simulink model "ADC_SPWM_Openloop_2_Version_2"  (R2024b)
settings: Solver=FixedStepDiscrete  StartTime=0.0  StopTime=inf  FixedStep=50e-6  RelTol=1e-3
model workspace (MAT data in the model file):
  f = 25
undefined symbols (not defined in the file): alpha, alpha_Lpf, C28x, CPU1, CPU2, DiscIntNeverNeededParam, Down, dspblkCoreblockFVToolHelper, Gain, gcbh, GPTRIP1SEL, T_period, Ts, TZ1, Up
libraries: c2802xlib x26, dspstat3 x8, c2837xDlib x2, c280xlib x2, simulink x1, mcbpositiondecoderlib x1, mcbcontrolslib x1
(part 2 of 2)

== system ADC_SPWM_Openloop_2_Version_2/If Action Subsystem ==
  In1 : Inport
  Action Port : ActionPort  ActionPortLabel=if(u1 > 0.005)
  Out1 : Outport
  wires:
  In1/1 -> Out1/1

== system ADC_SPWM_Openloop_2_Version_2/If Action Subsystem1 ==
  In1 : Inport
  Action Port : ActionPort  ActionPortLabel=else
  Gain : Gain  Gain=0
  Out1 : Outport
  wires:
  In1/1 -> Gain/1
  Gain/1 -> Out1/1

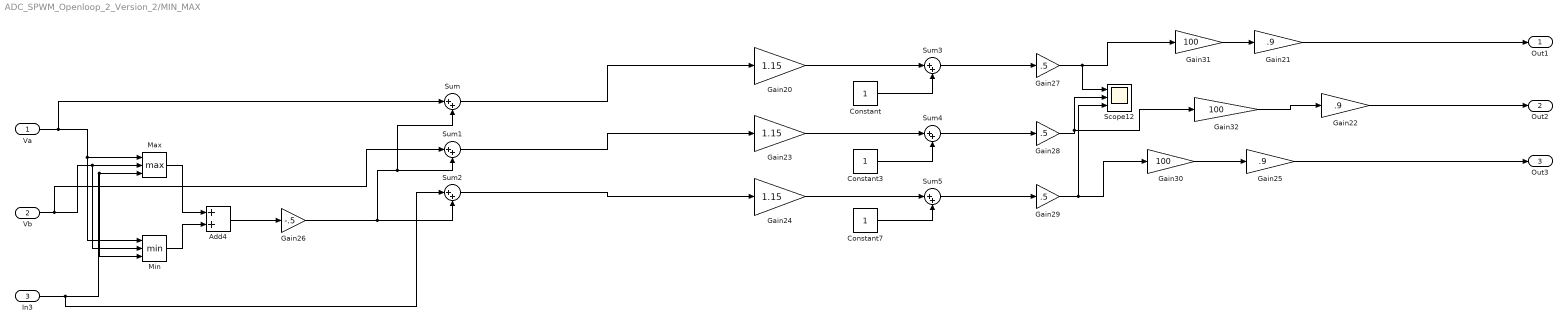
== system ADC_SPWM_Openloop_2_Version_2/MIN_MAX ==
  Va : Inport
  Vb : Inport  Port=2
  In3 : Inport  Port=3
  Add4 : Sum
  Constant : Constant
  Constant3 : Constant
  Constant7 : Constant
  Gain20 : Gain  Gain=1.15
  Gain21 : Gain  Gain=.9
  Gain22 : Gain  Gain=.9
  Gain23 : Gain  Gain=1.15
  Gain24 : Gain  Gain=1.15
  Gain25 : Gain  Gain=.9
  Gain26 : Gain  Gain=-.5
  Gain27 : Gain  Gain=.5
  Gain28 : Gain  Gain=.5
  Gain29 : Gain  Gain=.5
  Gain30 : Gain  Gain=100
  Gain31 : Gain  Gain=100
  Gain32 : Gain  Gain=100
  Max : MinMax  Function=max  Inputs=3
  Min : MinMax  Inputs=3
  Scope12 : Scope  NumInputPorts=3
  Sum{,1..5} (6 alike) : Sum  Inputs=|++
  Out1 : Outport
  Out2 : Outport  Port=2
  Out3 : Outport  Port=3
  wires:
  Gain28/1 -> Scope12/2, Gain32/1
  Sum3/1 -> Gain27/1
  Va/1 -> Sum/1, Min/1, Max/1
  Gain32/1 -> Gain22/1
  In3/1 -> Sum2/1, Min/3, Max/3
  Gain29/1 -> Scope12/3, Gain30/1
  Vb/1 -> Sum1/1, Min/2, Max/2
  Constant7/1 -> Sum5/2
  Sum/1 -> Gain20/1
  Gain26/1 -> Sum/2, Sum1/2, Sum2/2
  Add4/1 -> Gain26/1
  Gain30/1 -> Gain25/1
  Min/1 -> Add4/2
  Gain20/1 -> Sum3/1
  Gain27/1 -> Scope12/1, Gain31/1
  Constant3/1 -> Sum4/2
  Gain24/1 -> Sum5/1
  Constant/1 -> Sum3/2
  Sum4/1 -> Gain28/1
  Gain21/1 -> Out1/1
  Sum1/1 -> Gain23/1
  Max/1 -> Add4/1
  Gain25/1 -> Out3/1
  Gain31/1 -> Gain21/1
  Sum2/1 -> Gain24/1
  Gain23/1 -> Sum4/1
  Sum5/1 -> Gain29/1
  Gain22/1 -> Out2/1

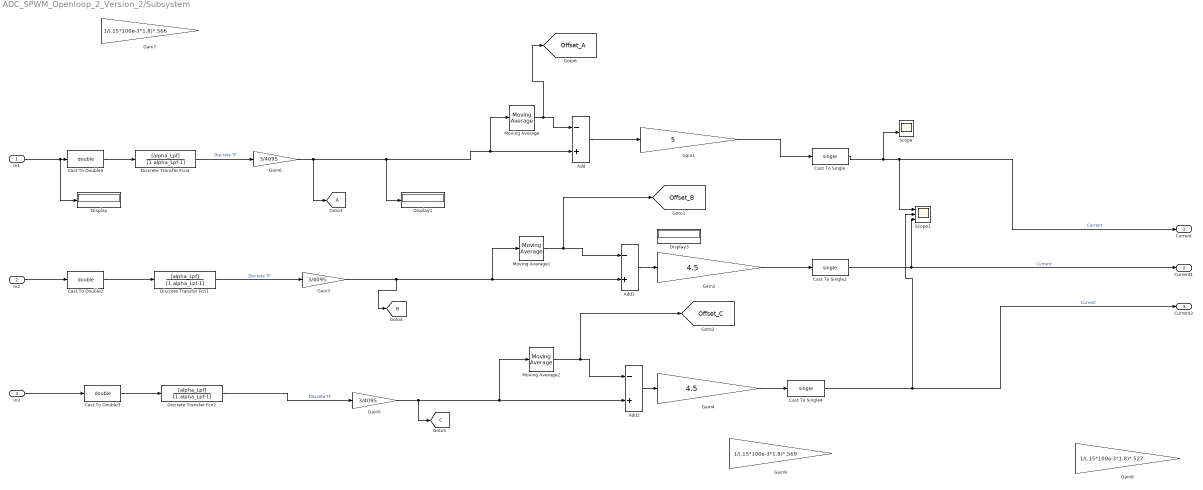
== system ADC_SPWM_Openloop_2_Version_2/Subsystem ==
  In1 : Inport
  In2 : Inport  Port=2
  In3 : Inport  Port=3
  Add : Sum  Inputs=-+
  Add1 : Sum  Inputs=-+
  Add2 : Sum  Inputs=-+
  Cast To Double2 : DataTypeConversion  OutDataTypeStr=double  SaturateOnIntegerOverflow=off  RndMeth=Floor
  Cast To Double3 : DataTypeConversion  OutDataTypeStr=double  SaturateOnIntegerOverflow=off  RndMeth=Floor
  Cast To Double5 : DataTypeConversion  OutDataTypeStr=double  SaturateOnIntegerOverflow=off  RndMeth=Floor
  Cast To Single : DataTypeConversion  OutDataTypeStr=single  SaturateOnIntegerOverflow=off  RndMeth=Floor
  Cast To Single2 : DataTypeConversion  OutDataTypeStr=single  SaturateOnIntegerOverflow=off  RndMeth=Floor
  Cast To Single4 : DataTypeConversion  OutDataTypeStr=single  SaturateOnIntegerOverflow=off  RndMeth=Floor
  Discrete Transfer Fcn1 : DiscreteTransferFcn  LoadFcn=dspblkCoreblockFVToolHelper(gcbh,'load');  Numerator=[alpha_Lpf]  Denominator=[1 alpha_Lpf-1]  InitialStates=1768/alpha_Lpf  RndMeth=Nearest
      settings: CopyFcn=dspblkCoreblockFVToolHelper(gcbh,'copy');  DeleteFcn=dspblkCoreblockFVToolHelper(gcbh,'close');  ModelCloseFcn=dspblkCoreblockFVToolHelper(gcbh,'close');  PreSaveFcn=dspblkCoreblockFVToolHelper(gcbh,'presave');  PostSaveFcn=dspblkCoreblockFVToolHelper(gcbh,'postsave');  CloseFcn=dspblkCoreblockFVToolHelper(gcbh,'close');
  Discrete Transfer Fcn2 : DiscreteTransferFcn  LoadFcn=dspblkCoreblockFVToolHelper(gcbh,'load');  Numerator=[alpha_Lpf]  Denominator=[1 alpha_Lpf-1]  InitialStates=1780/alpha_Lpf  RndMeth=Nearest
      settings: CopyFcn=dspblkCoreblockFVToolHelper(gcbh,'copy');  DeleteFcn=dspblkCoreblockFVToolHelper(gcbh,'close');  ModelCloseFcn=dspblkCoreblockFVToolHelper(gcbh,'close');  PreSaveFcn=dspblkCoreblockFVToolHelper(gcbh,'presave');  PostSaveFcn=dspblkCoreblockFVToolHelper(gcbh,'postsave');  CloseFcn=dspblkCoreblockFVToolHelper(gcbh,'close');
  Discrete Transfer Fcn4 : DiscreteTransferFcn  LoadFcn=dspblkCoreblockFVToolHelper(gcbh,'load');  Numerator=[alpha_Lpf]  Denominator=[1 alpha_Lpf-1]  InitialStates=1782/alpha_Lpf  RndMeth=Nearest
      settings: CopyFcn=dspblkCoreblockFVToolHelper(gcbh,'copy');  DeleteFcn=dspblkCoreblockFVToolHelper(gcbh,'close');  ModelCloseFcn=dspblkCoreblockFVToolHelper(gcbh,'close');  PreSaveFcn=dspblkCoreblockFVToolHelper(gcbh,'presave');  PostSaveFcn=dspblkCoreblockFVToolHelper(gcbh,'postsave');  CloseFcn=dspblkCoreblockFVToolHelper(gcbh,'close');
  Display : Display
  Display1 : Display
  Display3 : Display
  Gain1 : Gain  Gain=5
  Gain2 : Gain  Gain=4.5
  Gain3 : Gain  Gain=3/4095
  Gain4 : Gain  Gain=4.5
  Gain5 : Gain  Gain=3/4095
  Gain6 : Gain  Gain=3/4095
  Gain7 : Gain  Gain=1/(.15*100e-3*1.8)*.566
  Gain8 : Gain  Gain=1/(.15*100e-3*1.8)*.527
  Gain9 : Gain  Gain=1/(.15*100e-3*1.8)*.569
  Goto3 : Goto  TagVisibility=global
  Moving Average : dspstat3/Moving Average  Method=Exponential weighting  ForgettingFactorPort=off  SpecifyWindowLength=on  WindowLength=4  OverlapLength=3  AllowArbitraryInputLength=off  ForgettingFactor=0.99  SimulateUsing=Interpreted execution
  Moving Average1 : dspstat3/Moving Average  Method=Exponential weighting  ForgettingFactorPort=off  SpecifyWindowLength=on  WindowLength=4  OverlapLength=3  AllowArbitraryInputLength=off  ForgettingFactor=0.99  SimulateUsing=Interpreted execution
  Moving Average2 : dspstat3/Moving Average  Method=Exponential weighting  ForgettingFactorPort=off  SpecifyWindowLength=on  WindowLength=4  OverlapLength=3  AllowArbitraryInputLength=off  ForgettingFactor=0.99  SimulateUsing=Interpreted execution
  Scope : Scope  NumInputPorts=2
  Scope1 : Scope  NumInputPorts=3
  Current : Outport
  Current1 : Outport  Port=2
  Current2 : Outport  Port=3
  tag scope: B=global, C=global, Offset_A=global, Offset_B=global, Offset_C=global
  wires:
  Discrete Transfer Fcn4/1 -> Gain6/1  "Discrete TF"
  Cast To Double5/1 -> Discrete Transfer Fcn4/1
  Cast To Double3/1 -> Discrete Transfer Fcn2/1
  Cast To Double2/1 -> Discrete Transfer Fcn1/1
  Gain5/1 -> [C], Moving Average2/1, Add2/2
  Cast To Single4/1 -> Scope1/2, Current2/1  "Current"
  Add/1 -> Gain1/1
  Add1/1 -> Gain2/1
  Gain4/1 -> Cast To Single4/1
  Add2/1 -> Gain4/1
  Discrete Transfer Fcn1/1 -> Gain3/1  "Discrete TF"
  Discrete Transfer Fcn2/1 -> Gain5/1  "Discrete TF"
  In2/1 -> Cast To Double2/1
  In1/1 -> Display/1, Cast To Double5/1
  Gain2/1 -> Cast To Single2/1
  Cast To Single/1 -> Scope/2, Scope1/1, Current/1  "Current"
  Gain1/1 -> Cast To Single/1
  Gain6/1 -> Goto3/1, Moving Average/1, Add/2, Display1/1
  Cast To Single2/1 -> Scope1/3, Current1/1  "Current"
  In3/1 -> Cast To Double3/1
  Gain3/1 -> [B], Moving Average1/1, Add1/2
  Moving Average/1 -> [Offset_A], Add/1
  Moving Average1/1 -> [Offset_B], Add1/1
  Moving Average2/1 -> [Offset_C], Add2/1

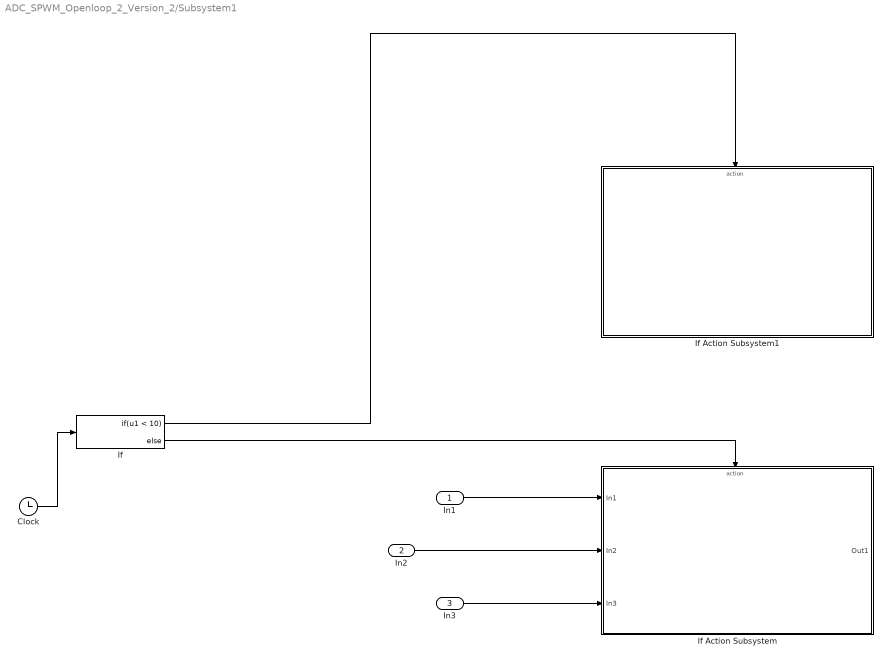
== system ADC_SPWM_Openloop_2_Version_2/Subsystem1 ==
  In1 : Inport
  In2 : Inport  Port=2
  In3 : Inport  Port=3
  Clock : Clock
  If : If  IfExpression=u1 < 10
  If Action Subsystem : Subsystem  TreatAsAtomicUnit=on
  If Action Subsystem1 : Subsystem  TreatAsAtomicUnit=on
  wires:
  Clock/1 -> If/1
  In1/1 -> If Action Subsystem/1(In1)
  In2/1 -> If Action Subsystem/2(In2)
  In3/1 -> If Action Subsystem/3(In3)
  If/1 -> If Action Subsystem1/Action
  If/2 -> If Action Subsystem/Action

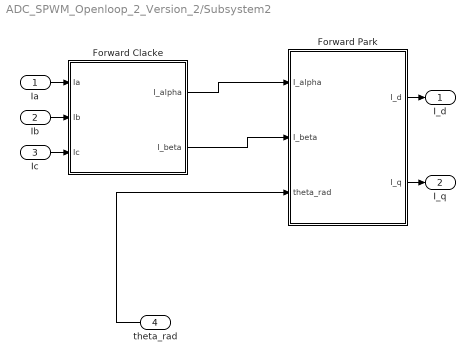
== system ADC_SPWM_Openloop_2_Version_2/Subsystem2 ==
  Ia : Inport
  Ib : Inport  Port=2
  Ic : Inport  Port=3
  theta_rad : Inport  Port=4
  Forward Clacke : Subsystem
  Forward Park : Subsystem
  I_d : Outport
  I_q : Outport  Port=2
  wires:
  Ic/1 -> Forward Clacke/3(Ic)
  Forward Clacke/2(I_beta) -> Forward Park/2(I_beta)
  Forward Clacke/1(I_alpha) -> Forward Park/1(I_alpha)
  Ia/1 -> Forward Clacke/1(Ia)
  Forward Park/1(I_d) -> I_d/1
  Forward Park/2(I_q) -> I_q/1
  Ib/1 -> Forward Clacke/2(Ib)
  theta_rad/1 -> Forward Park/3(theta_rad)

== system ADC_SPWM_Openloop_2_Version_2/Subsystem1/If Action Subsystem ==
  In1 : Inport
  In2 : Inport  Port=2
  In3 : Inport  Port=3
  Action Port : ActionPort  ActionPortLabel=else
  Out1 : Outport

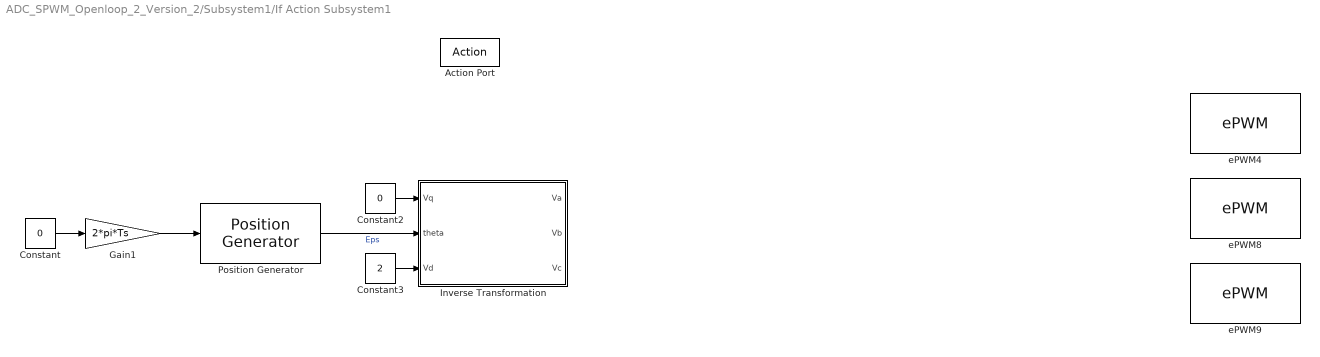
== system ADC_SPWM_Openloop_2_Version_2/Subsystem1/If Action Subsystem1 ==
  Action Port : ActionPort  ActionPortLabel=if(u1 < 10)
  Constant : Constant  Value=0
  Constant2 : Constant  Value=0
  Constant3 : Constant  Value=2
  Gain1 : Gain  Gain=2*pi*Ts
  Inverse Transformation : Subsystem
  Position Generator : mcbcontrolslib/Position Generator  AngleOutput=Radians  ExternalReset=none  Offset=0
      settings: LibrarySourceBlock=mcbhdllib/Controls/Control Reference/Position Generator
  ePWM4 : c2802xlib/ePWM  PwmType=C2000_Type4  useModule=ePWM1  ePWMxLINKTBPRD=Not Linked  periodUnits=Clock cycles  timerSource=Specify via dialog  timerPeriod_clk=Timer_period  timerPeriod_sec=0.0001  tbshadow=Counter equals to zero  countingMode=Up-Down  phaseActiveEnable=Disable  phaseDirection=Count down after sync  phaseActive=0  synchronizationEnable=off  dcaevt1Sync=off  dcbevt1Sync=off  synchronizationOption=Counter equals to zero (CTR=Zero)  dcbevt1SyncOut=off  dcaevt1SyncOut=off  cmpdSyncOut=off  cmpcSyncOut=off  cmpbSyncOut=off  zeroSyncOut=off  swfSyncOut=off  perSynchronizationOption=Counter equals to period (CTR=PRD)  clockPrescale=1  HSclockPrescale=1  enswap=off  ePWMxAStatus=on  ePWMxAactionLogic1=Do nothing  ePWMxAactionLogic2=Do nothing  ePWMxAactionLogic3=Clear  ePWMxAactionLogic4=Set  ePWMxAactionLogic5=Do nothing  ePWMxAactionLogic6=Do nothing  ePWMxACSFenable=off  ePWMxACSFvalue=Forcing disable  ePWMxASFreload=Zero  ePWMxBStatus=off  ePWMxBactionLogic1=Do nothing  ePWMxBactionLogic2=Do nothing  ePWMxBactionLogic3=Set  ePWMxBactionLogic4=Clear  ePWMxBactionLogic5=Do nothing  ePWMxBactionLogic6=Do nothing  ePWMxBCSFenable=off  ePWMxBCSFvalue=Forcing disable  ePWMxBSFreload=Zero  ePWNxBOutWay=off  ePWMxLINKCMPA=Not Linked  CMPAUnits=Percentages  CMPASource=Input port  CMPAValue_per=0  CMPAValue_clk=0  enCMPAshadow=Counter equals to zero (CTR=Zero)  ePWMxLINKCMPB=Not Linked  CMPBUnits=Clock cycles  CMPBSource=Specify via dialog  CMPBValue_per=50  CMPBValue_clk=32000  enCMPBshadow=Counter equals to zero (CTR=Zero)  ePWMxLINKCMPC=Not Linked  CMPCUnits=Clock cycles  CMPCSource=Specify via dialog  CMPCValue_per=50  CMPCValue_clk=32000  enCMPCshadow=Counter equals to zero (CTR=Zero)  ePWMxLINKCMPD=Not Linked  CMPDUnits=Clock cycles  CMPDSource=Specify via dialog  CMPDValue_per=50  CMPDValue_clk=32000  enCMPDshadow=Counter equals to zero (CTR=Zero)  enableDBePWMxA=on  enableDBePWMxB=on  enhalfcycle=off  DBpolarity=Active high complementary (AHC)  DBedgeDelay=Positive  DBSource_ePWMxA=ePWMxA  DBSource_ePWMxB=ePWMxA  DBPeriodUnits=Clock cycles  DBperiodSource=Specify via dialog  REDperiod=100  FEDperiod=100  REDperiod_sec=0  FEDperiod_sec=0  LoadModeDBRED=Immediate without using shadow  LoadModeDBFED=Immediate without using shadow  adcstartModuleA=on  adcrequestEventA=First event  adcstartEventA=Digital Compare Module A Event 1 start of conversion (DCAEVT1.soc)  adcstartEventA_type2=Counter equals to period (CTR=PRD)  adcstartModuleB=off  adcrequestEventB=First event  adcstartEventB=Counter equals to zero (CTR=Zero)  adcstartEventB_type2=Counter equals to zero (CTR=Zero)  intEn=on  intPrd=First event  intSel=Counter equals to zero (CTR=Zero)  intSel_type2=Counter equals to period (CTR=PRD)  hrpe=off  enHRPWM=off  HRPWM_LoadMode=Counter equals to period (CTR=PRD)  HRPWM_CTLMode=Duty or Period control mode  HRPWM_EDGMode=Both edge  hrpeb=off  enHRPWMB=off  HRPWM_LoadModeB=Counter equals to zero (CTR=ZERO)  HRPWM_CTLModeB=Duty or Period control mode  HRPWM_EDGModeB=Both edge  enHRDBRED=off  enHRDBFED=off  enSFO=on  enautoconv=on  chopperEnable=off  chopperFrequency=1  chopperFirstwidth=1  chopperDuty=12.5%  tripZonesource=Specify via dialog  tzselOSHT1=off  tzselOSHT2=off  tzselOSHT3=off  tzselOSHT4=off  tzselOSHT5=off  tzselOSHT6=off  tzselOSHDCAEV1=off  tzselOSHDCBEV1=off  tzselCBC1=off  tzselCBC2=off  tzselCBC3=off  tzselCBC4=off  tzselCBC5=off  tzselCBC6=off  tzselCBCDCAEV2=off  tzselCBCDCBEV2=off  enTzOstIntr=off  enTzCbcIntr=off  enTzDCAEVT1Intr=off  enTzDCAEVT2Intr=off  enTzDCBEVT1Intr=off  enTzDCBEVT2Intr=off  tzclrCBCLatch=Counter equals to zero (CTR=Zero)  ePWMxAforced=No action  ePWMxBforced=No action  DCAEVT1forced=No action  DCBEVT1forced=No action  DCAEVT2forced=No action  DCBEVT2forced=No action  dcah=Trip Zone 1 input (TZ1)  dcal=Trip Zone 2 input (TZ2)  dcbh=Trip Zone 1 input (TZ1)  dcbl=Trip Zone 2 input (TZ2)  dcah_type2=GPTRIP1SEL/(TZ1)  dcal_type2=GPTRIP1SEL/(TZ1)  dcbh_type2=GPTRIP1SEL/(TZ1)  dcbl_type2=GPTRIP1SEL/(TZ1)  gendcaevt1=Event disabled  gendcaevt2=Event disabled  gendcbevt1=Event disabled  gendcbevt2=Event disabled  dcaevt1src=DCAEVT1 with sync  dcaevt2src=DCAEVT2 with sync  dcbevt1src=DCBEVT1 with sync  dcbevt2src=DCBEVT2 with sync  pulsesel=Counter equals to zero (CTR=Zero)  blankinv=off  blankoffset=0  blankwidth=0  evsrcsel=Filtered version of DCAEVT1 (DCAEVT1FILT)  encape=off
      settings: LibrarySourceBlock=c2837xDlib/ePWM
  ePWM8 : c2802xlib/ePWM  PwmType=C2000_Type4  useModule=ePWM2  ePWMxLINKTBPRD=Not Linked  periodUnits=Clock cycles  timerSource=Specify via dialog  timerPeriod_clk=Timer_period  timerPeriod_sec=0.0001  tbshadow=Counter equals to zero  countingMode=Up-Down  phaseActiveEnable=Disable  phaseDirection=Count down after sync  phaseActive=0  synchronizationEnable=off  dcaevt1Sync=off  dcbevt1Sync=off  synchronizationOption=Disable  dcbevt1SyncOut=off  dcaevt1SyncOut=off  cmpdSyncOut=off  cmpcSyncOut=off  cmpbSyncOut=off  zeroSyncOut=off  swfSyncOut=off  perSynchronizationOption=Counter equals to period (CTR=PRD)  clockPrescale=1  HSclockPrescale=1  enswap=off  ePWMxAStatus=on  ePWMxAactionLogic1=Do nothing  ePWMxAactionLogic2=Do nothing  ePWMxAactionLogic3=Clear  ePWMxAactionLogic4=Set  ePWMxAactionLogic5=Do nothing  ePWMxAactionLogic6=Do nothing  ePWMxACSFenable=off  ePWMxACSFvalue=Forcing disable  ePWMxASFreload=Zero  ePWMxBStatus=on  ePWMxBactionLogic1=Do nothing  ePWMxBactionLogic2=Do nothing  ePWMxBactionLogic3=Set  ePWMxBactionLogic4=Clear  ePWMxBactionLogic5=Do nothing  ePWMxBactionLogic6=Do nothing  ePWMxBCSFenable=off  ePWMxBCSFvalue=Forcing disable  ePWMxBSFreload=Zero  ePWNxBOutWay=off  ePWMxLINKCMPA=Not Linked  CMPAUnits=Percentages  CMPASource=Input port  CMPAValue_per=0  CMPAValue_clk=0  enCMPAshadow=Counter equals to zero (CTR=Zero)  ePWMxLINKCMPB=Not Linked  CMPBUnits=Clock cycles  CMPBSource=Specify via dialog  CMPBValue_per=50  CMPBValue_clk=32000  enCMPBshadow=Counter equals to zero (CTR=Zero)  ePWMxLINKCMPC=Not Linked  CMPCUnits=Clock cycles  CMPCSource=Specify via dialog  CMPCValue_per=50  CMPCValue_clk=32000  enCMPCshadow=Counter equals to zero (CTR=Zero)  ePWMxLINKCMPD=Not Linked  CMPDUnits=Clock cycles  CMPDSource=Specify via dialog  CMPDValue_per=50  CMPDValue_clk=32000  enCMPDshadow=Counter equals to zero (CTR=Zero)  enableDBePWMxA=on  enableDBePWMxB=on  enhalfcycle=off  DBpolarity=Active high complementary (AHC)  DBedgeDelay=Positive  DBSource_ePWMxA=ePWMxA  DBSource_ePWMxB=ePWMxA  DBPeriodUnits=Clock cycles  DBperiodSource=Specify via dialog  REDperiod=400  FEDperiod=400  REDperiod_sec=0  FEDperiod_sec=0  LoadModeDBRED=Immediate without using shadow  LoadModeDBFED=Immediate without using shadow  adcstartModuleA=on  adcrequestEventA=First event  adcstartEventA=Digital Compare Module A Event 1 start of conversion (DCAEVT1.soc)  adcstartEventA_type2=Counter equals to period (CTR=PRD)  adcstartModuleB=off  adcrequestEventB=First event  adcstartEventB=Counter equals to zero (CTR=Zero)  adcstartEventB_type2=Counter equals to zero (CTR=Zero)  intEn=on  intPrd=First event  intSel=Counter equals to zero (CTR=Zero)  intSel_type2=Counter equals to period (CTR=PRD)  hrpe=off  enHRPWM=off  HRPWM_LoadMode=Counter equals to period (CTR=PRD)  HRPWM_CTLMode=Duty or Period control mode  HRPWM_EDGMode=Both edge  hrpeb=off  enHRPWMB=off  HRPWM_LoadModeB=Counter equals to zero (CTR=ZERO)  HRPWM_CTLModeB=Duty or Period control mode  HRPWM_EDGModeB=Both edge  enHRDBRED=off  enHRDBFED=off  enSFO=on  enautoconv=on  chopperEnable=off  chopperFrequency=1  chopperFirstwidth=1  chopperDuty=12.5%  tripZonesource=Specify via dialog  tzselOSHT1=off  tzselOSHT2=off  tzselOSHT3=off  tzselOSHT4=off  tzselOSHT5=off  tzselOSHT6=off  tzselOSHDCAEV1=off  tzselOSHDCBEV1=off  tzselCBC1=off  tzselCBC2=off  tzselCBC3=off  tzselCBC4=off  tzselCBC5=off  tzselCBC6=off  tzselCBCDCAEV2=off  tzselCBCDCBEV2=off  enTzOstIntr=off  enTzCbcIntr=off  enTzDCAEVT1Intr=off  enTzDCAEVT2Intr=off  enTzDCBEVT1Intr=off  enTzDCBEVT2Intr=off  tzclrCBCLatch=Counter equals to zero (CTR=Zero)  ePWMxAforced=No action  ePWMxBforced=No action  DCAEVT1forced=No action  DCBEVT1forced=No action  DCAEVT2forced=No action  DCBEVT2forced=No action  dcah=Trip Zone 1 input (TZ1)  dcal=Trip Zone 2 input (TZ2)  dcbh=Trip Zone 1 input (TZ1)  dcbl=Trip Zone 2 input (TZ2)  dcah_type2=GPTRIP1SEL/(TZ1)  dcal_type2=GPTRIP1SEL/(TZ1)  dcbh_type2=GPTRIP1SEL/(TZ1)  dcbl_type2=GPTRIP1SEL/(TZ1)  gendcaevt1=Event disabled  gendcaevt2=Event disabled  gendcbevt1=Event disabled  gendcbevt2=Event disabled  dcaevt1src=DCAEVT1 with sync  dcaevt2src=DCAEVT2 with sync  dcbevt1src=DCBEVT1 with sync  dcbevt2src=DCBEVT2 with sync  pulsesel=Counter equals to zero (CTR=Zero)  blankinv=off  blankoffset=0  blankwidth=0  evsrcsel=Filtered version of DCAEVT1 (DCAEVT1FILT)  encape=off
      settings: LibrarySourceBlock=c2837xDlib/ePWM
  ePWM9 : c2802xlib/ePWM  PwmType=C2000_Type4  useModule=ePWM4  ePWMxLINKTBPRD=Not Linked  periodUnits=Clock cycles  timerSource=Specify via dialog  timerPeriod_clk=Timer_period  timerPeriod_sec=0.0001  tbshadow=Counter equals to zero  countingMode=Up-Down  phaseActiveEnable=Disable  phaseDirection=Count down after sync  phaseActive=0  synchronizationEnable=off  dcaevt1Sync=off  dcbevt1Sync=off  synchronizationOption=Disable  dcbevt1SyncOut=off  dcaevt1SyncOut=off  cmpdSyncOut=off  cmpcSyncOut=off  cmpbSyncOut=off  zeroSyncOut=off  swfSyncOut=off  perSynchronizationOption=Counter equals to period (CTR=PRD)  clockPrescale=1  HSclockPrescale=1  enswap=off  ePWMxAStatus=on  ePWMxAactionLogic1=Do nothing  ePWMxAactionLogic2=Do nothing  ePWMxAactionLogic3=Clear  ePWMxAactionLogic4=Set  ePWMxAactionLogic5=Do nothing  ePWMxAactionLogic6=Do nothing  ePWMxACSFenable=off  ePWMxACSFvalue=Forcing disable  ePWMxASFreload=Zero  ePWMxBStatus=on  ePWMxBactionLogic1=Do nothing  ePWMxBactionLogic2=Do nothing  ePWMxBactionLogic3=Set  ePWMxBactionLogic4=Clear  ePWMxBactionLogic5=Do nothing  ePWMxBactionLogic6=Do nothing  ePWMxBCSFenable=off  ePWMxBCSFvalue=Forcing disable  ePWMxBSFreload=Zero  ePWNxBOutWay=off  ePWMxLINKCMPA=Not Linked  CMPAUnits=Percentages  CMPASource=Input port  CMPAValue_per=0  CMPAValue_clk=0  enCMPAshadow=Counter equals to zero (CTR=Zero)  ePWMxLINKCMPB=Not Linked  CMPBUnits=Clock cycles  CMPBSource=Specify via dialog  CMPBValue_per=50  CMPBValue_clk=32000  enCMPBshadow=Counter equals to zero (CTR=Zero)  ePWMxLINKCMPC=Not Linked  CMPCUnits=Clock cycles  CMPCSource=Specify via dialog  CMPCValue_per=50  CMPCValue_clk=32000  enCMPCshadow=Counter equals to zero (CTR=Zero)  ePWMxLINKCMPD=Not Linked  CMPDUnits=Clock cycles  CMPDSource=Specify via dialog  CMPDValue_per=50  CMPDValue_clk=32000  enCMPDshadow=Counter equals to zero (CTR=Zero)  enableDBePWMxA=on  enableDBePWMxB=on  enhalfcycle=off  DBpolarity=Active high complementary (AHC)  DBedgeDelay=Positive  DBSource_ePWMxA=ePWMxA  DBSource_ePWMxB=ePWMxA  DBPeriodUnits=Clock cycles  DBperiodSource=Specify via dialog  REDperiod=400  FEDperiod=400  REDperiod_sec=0  FEDperiod_sec=0  LoadModeDBRED=Immediate without using shadow  LoadModeDBFED=Immediate without using shadow  adcstartModuleA=on  adcrequestEventA=First event  adcstartEventA=Digital Compare Module A Event 1 start of conversion (DCAEVT1.soc)  adcstartEventA_type2=Counter equals to period (CTR=PRD)  adcstartModuleB=off  adcrequestEventB=First event  adcstartEventB=Counter equals to zero (CTR=Zero)  adcstartEventB_type2=Counter equals to zero (CTR=Zero)  intEn=on  intPrd=First event  intSel=Counter equals to zero (CTR=Zero)  intSel_type2=Counter equals to period (CTR=PRD)  hrpe=off  enHRPWM=off  HRPWM_LoadMode=Counter equals to period (CTR=PRD)  HRPWM_CTLMode=Duty or Period control mode  HRPWM_EDGMode=Both edge  hrpeb=off  enHRPWMB=off  HRPWM_LoadModeB=Counter equals to zero (CTR=ZERO)  HRPWM_CTLModeB=Duty or Period control mode  HRPWM_EDGModeB=Both edge  enHRDBRED=off  enHRDBFED=off  enSFO=on  enautoconv=on  chopperEnable=off  chopperFrequency=1  chopperFirstwidth=1  chopperDuty=12.5%  tripZonesource=Specify via dialog  tzselOSHT1=off  tzselOSHT2=off  tzselOSHT3=off  tzselOSHT4=off  tzselOSHT5=off  tzselOSHT6=off  tzselOSHDCAEV1=off  tzselOSHDCBEV1=off  tzselCBC1=off  tzselCBC2=off  tzselCBC3=off  tzselCBC4=off  tzselCBC5=off  tzselCBC6=off  tzselCBCDCAEV2=off  tzselCBCDCBEV2=off  enTzOstIntr=off  enTzCbcIntr=off  enTzDCAEVT1Intr=off  enTzDCAEVT2Intr=off  enTzDCBEVT1Intr=off  enTzDCBEVT2Intr=off  tzclrCBCLatch=Counter equals to zero (CTR=Zero)  ePWMxAforced=No action  ePWMxBforced=No action  DCAEVT1forced=No action  DCBEVT1forced=No action  DCAEVT2forced=No action  DCBEVT2forced=No action  dcah=Trip Zone 1 input (TZ1)  dcal=Trip Zone 2 input (TZ2)  dcbh=Trip Zone 1 input (TZ1)  dcbl=Trip Zone 2 input (TZ2)  dcah_type2=GPTRIP1SEL/(TZ1)  dcal_type2=GPTRIP1SEL/(TZ1)  dcbh_type2=GPTRIP1SEL/(TZ1)  dcbl_type2=GPTRIP1SEL/(TZ1)  gendcaevt1=Event disabled  gendcaevt2=Event disabled  gendcbevt1=Event disabled  gendcbevt2=Event disabled  dcaevt1src=DCAEVT1 with sync  dcaevt2src=DCAEVT2 with sync  dcbevt1src=DCBEVT1 with sync  dcbevt2src=DCBEVT2 with sync  pulsesel=Counter equals to zero (CTR=Zero)  blankinv=off  blankoffset=0  blankwidth=0  evsrcsel=Filtered version of DCAEVT1 (DCAEVT1FILT)  encape=off
      settings: LibrarySourceBlock=c2837xDlib/ePWM
  wires:
  Constant/1 -> Gain1/1
  Constant3/1 -> Inverse Transformation/3(Vd)
  Position Generator/1 -> Inverse Transformation/2(theta)  "Eps"
  Gain1/1 -> Position Generator/1
  Constant2/1 -> Inverse Transformation/1(Vq)

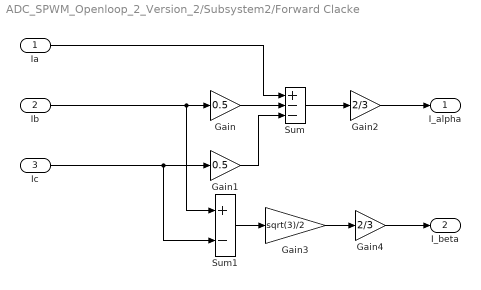
== system ADC_SPWM_Openloop_2_Version_2/Subsystem2/Forward Clacke ==
  Ia : Inport
  Ib : Inport  Port=2
  Ic : Inport  Port=3
  Gain : Gain  Gain=0.5
  Gain1 : Gain  Gain=0.5
  Gain2 : Gain  Gain=2/3
  Gain3 : Gain  Gain=sqrt(3)/2
  Gain4 : Gain  Gain=2/3
  Sum : Sum  Inputs=+--
  Sum1 : Sum  Inputs=+-
  I_alpha : Outport
  I_beta : Outport  Port=2
  wires:
  Ib/1 -> Gain/1, Sum1/1
  Gain/1 -> Sum/2
  Gain2/1 -> I_alpha/1
  Sum1/1 -> Gain3/1
  Gain1/1 -> Sum/3
  Ic/1 -> Gain1/1, Sum1/2
  Sum/1 -> Gain2/1
  Gain3/1 -> Gain4/1
  Ia/1 -> Sum/1
  Gain4/1 -> I_beta/1

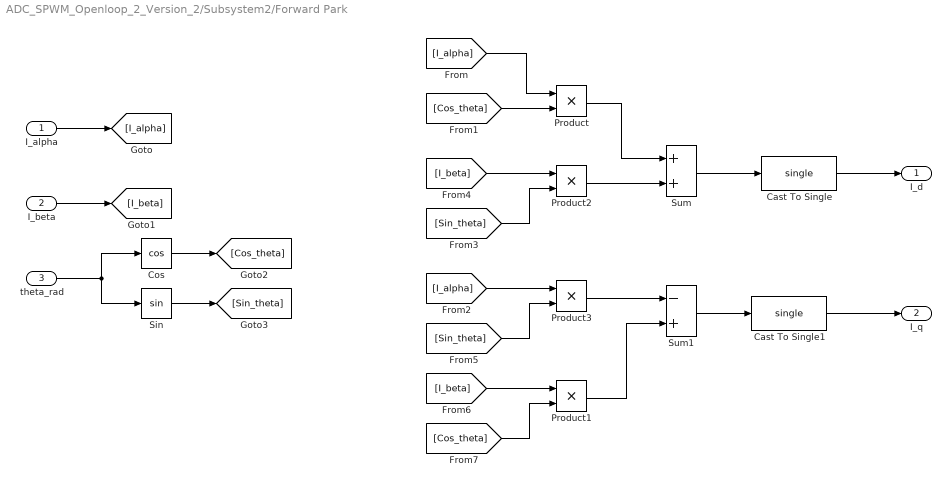
== system ADC_SPWM_Openloop_2_Version_2/Subsystem2/Forward Park ==
  I_alpha : Inport
  I_beta : Inport  Port=2
  theta_rad : Inport  Port=3
  Cast To Single : DataTypeConversion  OutDataTypeStr=single  SaturateOnIntegerOverflow=off  RndMeth=Floor
  Cast To Single1 : DataTypeConversion  OutDataTypeStr=single  SaturateOnIntegerOverflow=off  RndMeth=Floor
  Cos : Trigonometry  Operator=cos
  Product{,1..3} (4 alike) : Product
  Sin : Trigonometry
  Sum : Sum
  Sum1 : Sum  Inputs=-+
  I_d : Outport
  I_q : Outport  Port=2
  wires:
  [Cos_theta] -> Product1/2
  [I_beta] -> Product1/1
  [Sin_theta] -> Product3/2
  [I_alpha] -> Product3/1
  Product1/1 -> Sum1/2
  [I_beta] -> Product2/1
  [Sin_theta] -> Product2/2
  [Cos_theta] -> Product/2
  Sin/1 -> [Sin_theta]
  Cos/1 -> [Cos_theta]
  theta_rad/1 -> Cos/1, Sin/1
  [I_alpha] -> Product/1
  I_beta/1 -> [I_beta]
  I_alpha/1 -> [I_alpha]
  Product3/1 -> Sum1/1
  Product2/1 -> Sum/2
  Product/1 -> Sum/1
  Sum1/1 -> Cast To Single1/1
  Sum/1 -> Cast To Single/1
  Cast To Single/1 -> I_d/1
  Cast To Single1/1 -> I_q/1

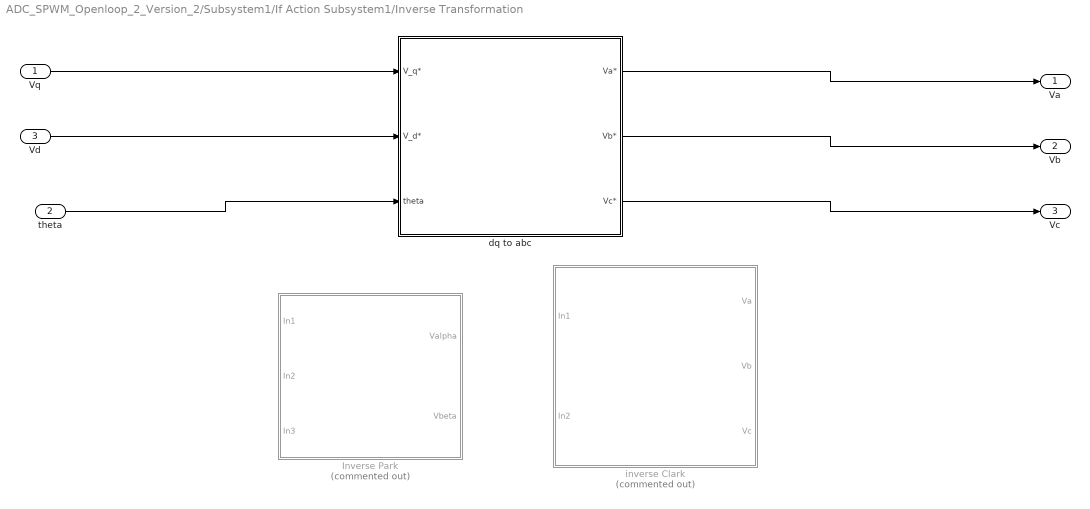
== system ADC_SPWM_Openloop_2_Version_2/Subsystem1/If Action Subsystem1/Inverse Transformation ==
  Vq : Inport
  theta : Inport  Port=2
  Vd : Inport  Port=3
  "Inverse Park " : Subsystem  Commented=on
  dq to abc : Subsystem
  inverse Clark : Subsystem  Commented=on
  Va : Outport
  Vb : Outport  Port=2
  Vc : Outport  Port=3
  wires:
  theta/1 -> dq to abc/3(theta)
  Vq/1 -> dq to abc/1(V_q*)
  Vd/1 -> dq to abc/2(V_d*)
  dq to abc/1(Va*) -> Va/1
  dq to abc/2(Vb*) -> Vb/1
  dq to abc/3(Vc*) -> Vc/1

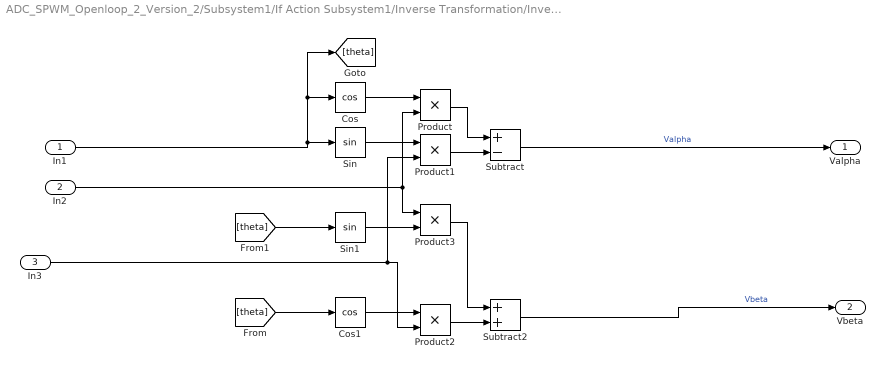
== system ADC_SPWM_Openloop_2_Version_2/Subsystem1/If Action Subsystem1/Inverse Transformation/Inverse Park  ==
  In1 : Inport
  In2 : Inport  Port=2
  In3 : Inport  Port=3
  Cos : Trigonometry  Operator=cos
  Cos1 : Trigonometry  Operator=cos
  Product{,1..3} (4 alike) : Product
  Sin : Trigonometry
  Sin1 : Trigonometry
  Subtract : Sum  Inputs=+-
  Subtract2 : Sum
  Valpha : Outport
  Vbeta : Outport  Port=2
  wires:
  Product3/1 -> Subtract2/1
  In3/1 -> Product2/2, Product1/2
  In1/1 -> Cos/1, [theta], Sin/1
  Subtract/1 -> Valpha/1  "Valpha"
  Product/1 -> Subtract/1
  Subtract2/1 -> Vbeta/1  "Vbeta"
  Product2/1 -> Subtract2/2
  Cos/1 -> Product/1
  Product1/1 -> Subtract/2
  [theta] -> Cos1/1
  In2/1 -> Product/2, Product3/1
  [theta] -> Sin1/1
  Sin/1 -> Product1/1
  Cos1/1 -> Product2/1
  Sin1/1 -> Product3/2

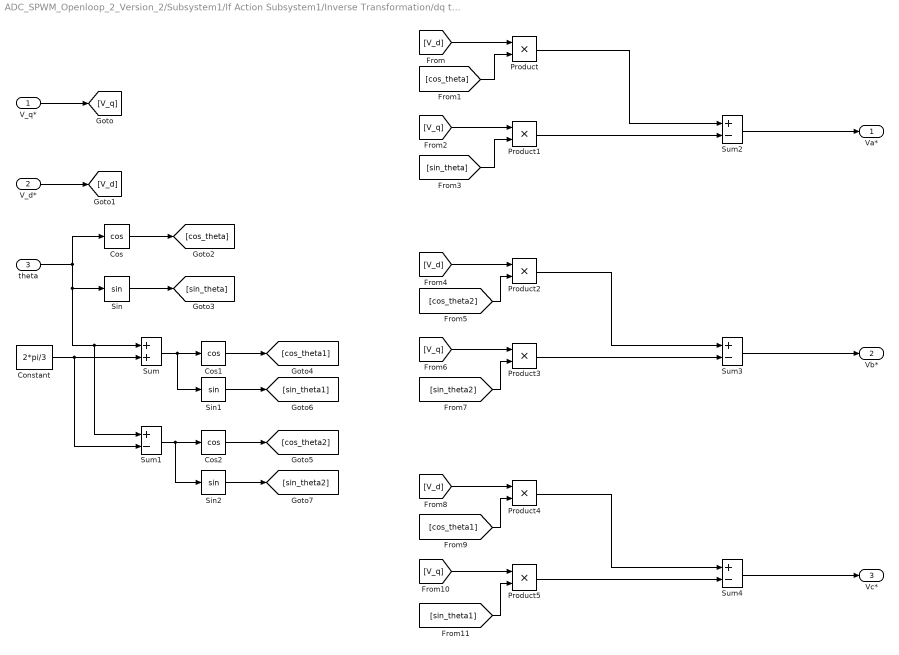
== system ADC_SPWM_Openloop_2_Version_2/Subsystem1/If Action Subsystem1/Inverse Transformation/dq to abc ==
  V_q* : Inport
  V_d* : Inport  Port=2
  theta : Inport  Port=3
  Constant : Constant  Value=2*pi/3
  Cos : Trigonometry  Operator=cos
  Cos1 : Trigonometry  Operator=cos
  Cos2 : Trigonometry  Operator=cos
  Product{,1..5} (6 alike) : Product
  Sin : Trigonometry
  Sin1 : Trigonometry
  Sin2 : Trigonometry
  Sum : Sum
  Sum{1..4} (4 alike) : Sum  Inputs=+-
  Va* : Outport
  Vb* : Outport  Port=2
  Vc* : Outport  Port=3
  wires:
  [sin_theta1] -> Product5/2
  [V_q] -> Product5/1
  [cos_theta1] -> Product4/2
  [V_d] -> Product4/1
  Product4/1 -> Sum4/1
  Product5/1 -> Sum4/2
  Sum4/1 -> Vc*/1
  [sin_theta2] -> Product3/2
  Sin2/1 -> [sin_theta2]
  Sin1/1 -> [sin_theta1]
  [V_q] -> Product3/1
  [cos_theta2] -> Product2/2
  [V_d] -> Product2/1
  Sum3/1 -> Vb*/1
  Product3/1 -> Sum3/2
  Product2/1 -> Sum3/1
  [sin_theta] -> Product1/2
  [V_q] -> Product1/1
  [cos_theta] -> Product/2
  [V_d] -> Product/1
  Product/1 -> Sum2/1
  Product1/1 -> Sum2/2
  Sum2/1 -> Va*/1
  Cos2/1 -> [cos_theta2]
  Cos1/1 -> [cos_theta1]
  Sum1/1 -> Cos2/1, Sin2/1
  Sum/1 -> Cos1/1, Sin1/1
  Constant/1 -> Sum/2, Sum1/2
  Sin/1 -> [sin_theta]
  Cos/1 -> [cos_theta]
  theta/1 -> Cos/1, Sin/1, Sum1/1, Sum/1
  V_d*/1 -> [V_d]
  V_q*/1 -> [V_q]

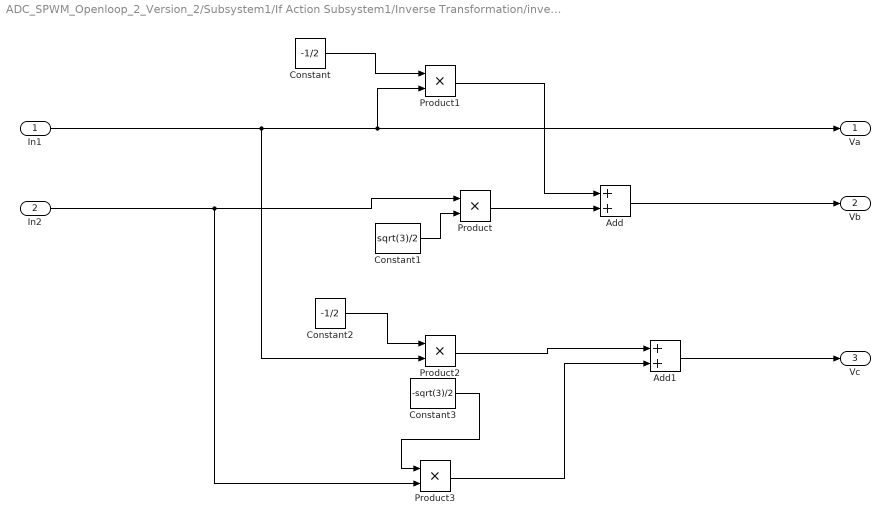
== system ADC_SPWM_Openloop_2_Version_2/Subsystem1/If Action Subsystem1/Inverse Transformation/inverse Clark ==
  In1 : Inport
  In2 : Inport  Port=2
  Add : Sum
  Add1 : Sum
  Constant : Constant  Value=-1/2
  Constant1 : Constant  Value=sqrt(3)/2
  Constant2 : Constant  Value=-1/2
  Constant3 : Constant  Value=-sqrt(3)/2
  Product{,1..3} (4 alike) : Product
  Va : Outport
  Vb : Outport  Port=2
  Vc : Outport  Port=3
  wires:
  In1/1 -> Va/1, Product1/2, Product2/2
  In2/1 -> Product/1, Product3/2
  Add/1 -> Vb/1
  Product3/1 -> Add1/2
  Constant/1 -> Product1/1
  Constant2/1 -> Product2/1
  Product/1 -> Add/2
  Constant1/1 -> Product/2
  Product1/1 -> Add/1
  Product2/1 -> Add1/1
  Add1/1 -> Vc/1
  Constant3/1 -> Product3/1

== matlab function ADC_SPWM_Openloop_2_Version_2/MATLAB Function1 ==
  data: u input; y output; f input; Ts input; numPeriods input
function y = dcOffset_longWindow(u, f, Ts, numPeriods)
% u            : input signal (sine wave + offset)
% f            : frequency of the sine wave (Hz)
% Ts           : sample time (s)
% numPeriods   : number of periods to average over (e.g., 10)
% y            : output = DC offset (running average from first sample)

persistent buffer sumBuf idx N count

if isempty(N)
    samplesPerPeriod = round(1 / (f * Ts));
    N = samplesPerPeriod * numPeriods;   % total window length
    buffer = zeros(N, 1);
    sumBuf = 0;
    idx = 1;
    count = 0;          % number of samples received so far
end

% Update circular buffer: subtract oldest only if buffer is already full
if count >= N
    % Full window mode: subtract the sample that will be overwritten
    sumBuf = sumBuf - buffer(idx);
else
    % Startup mode: no subtraction, just accumulating
    % (buffer initially zeros, so subtracting would incorrectly remove zeros)
end

% Store new sample and update sum
buffer(idx) = u;
sumBuf = sumBuf + u;
idx = mod(idx, N) + 1;
count = count + 1;

% Output the average over the actual number of samples received so far
if count < N
    y = sumBuf / count;    % running average from first sample
else
    y = sumBuf / N;        % steady-state full‑window average
end
end

== matlab function ADC_SPWM_Openloop_2_Version_2/MATLAB Function ==
  data: theta input; speed_rad_s output; Ts input
function speed_rad_s = calculate_speed(theta, Ts)
    % persistent variable remembers the angle from the previous time step
    persistent theta_prev;
    if isempty(theta_prev)
        theta_prev = 0;
    end

    % Calculate the raw delta
    delta_theta = theta - theta_prev;

    % UNWRAP LOGIC: Fix the jump from 2*pi to 0 (and vice versa)
    if delta_theta < -pi
        delta_theta = delta_theta + 2*pi;
    elseif delta_theta > pi
        delta_theta = delta_theta - 2*pi;
    end

    % Calculate speed and update previous value
    speed_rad_s = delta_theta / Ts;
    theta_prev = theta;
end

== matlab function ADC_SPWM_Openloop_2_Version_2/MATLAB Function2 ==
  data: u input; offset output; f input; Ts input; numPeriods input
function offset = dcOffset_Tracker(u, f, Ts, numPeriods)
%#codegen
% Speed-Adaptive DC Offset Tracker (Exponential Moving Average)
% OPTIMIZED FOR 4.5 kHz CONTROL LOOPS (Strict Single-Precision)

persistent y_prev

% --- 1. Strict Float Conversion ---
u_float = single(u);
f_float = single(f);
Ts_float = single(Ts);
numP_float = single(numPeriods);

% --- 2. Bumpless Initialization ---
if isempty(y_prev)
    y_prev = u_float; 
end

% --- 3. Safe Frequency Handling ---
f_abs = abs(f_float);

% Use single(2.0) to prevent double-precision math promotion!
f_min = single(2.0); 
if f_abs < f_min
    f_effective = f_min;
else
    f_effective = f_abs;
end

% --- 4. Calculate Alpha (Safe Math) ---
safe_numPeriods = max(numP_float, single(0.1)); 
alpha = (f_effective * Ts_float) / safe_numPeriods;

% --- 5. Alpha Bounds (High-Speed Safety) ---
if alpha > single(0.5)
    alpha = single(0.5);
end

% --- 6. Filter Update (Numerically Stable) ---
offset = y_prev + alpha * (u_float - y_prev);

% Store for the next cycle
y_prev = offset;

end

== matlab function ADC_SPWM_Openloop_2_Version_2/MATLAB Function3 ==
  data: u input; y output; f input; Ts input; numPeriods input
function y = dcOffset_longWindow(u, f, Ts, numPeriods)
% u            : input signal (sine wave + offset)
% f            : frequency of the sine wave (Hz)
% Ts           : sample time (s)
% numPeriods   : number of periods to average over (e.g., 10)
% y            : output = DC offset (running average from first sample)

persistent buffer sumBuf idx N count

if isempty(N)
    samplesPerPeriod = round(1 / (f * Ts));
    N = samplesPerPeriod * numPeriods;   % total window length
    buffer = zeros(N, 1);
    sumBuf = 0;
    idx = 1;
    count = 0;          % number of samples received so far
end

% Update circular buffer: subtract oldest only if buffer is already full
if count >= N
    % Full window mode: subtract the sample that will be overwritten
    sumBuf = sumBuf - buffer(idx);
else
    % Startup mode: no subtraction, just accumulating
    % (buffer initially zeros, so subtracting would incorrectly remove zeros)
end

% Store new sample and update sum
buffer(idx) = u;
sumBuf = sumBuf + u;
idx = mod(idx, N) + 1;
count = count + 1;

% Output the average over the actual number of samples received so far
if count < N
    y = sumBuf / count;    % running average from first sample
else
    y = sumBuf / N;        % steady-state full‑window average
end
end

== matlab function ADC_SPWM_Openloop_2_Version_2/MATLAB Function8 ==
  data: u input; y output; f input; Ts input; numPeriods input
function y = dcOffset_EMA(u, f, Ts, numPeriods)
%#codegen
% Exponential moving average - C-friendly
% Time constant = numPeriods * (1/f)

persistent alpha y_prev

if isempty(alpha)
    samplesPerPeriod = round(1 / (f * Ts));
    N = samplesPerPeriod * numPeriods;
    alpha = 1 / N;
    y_prev = u;
end

% First-order low-pass filter
y = y_prev + alpha * (u - y_prev);
y_prev = y;
end

== matlab function ADC_SPWM_Openloop_2_Version_2/MATLAB Function4 ==
  data: u input; y output; f input; Ts input; numPeriods input
function y = dcOffset_longWindow(u, f, Ts, numPeriods)
% u            : input signal (sine wave + offset)
% f            : frequency of the sine wave (Hz)
% Ts           : sample time (s)
% numPeriods   : number of periods to average over (e.g., 10)
% y            : output = DC offset (running average from first sample)

persistent buffer sumBuf idx N count

if isempty(N)
    samplesPerPeriod = round(1 / (f * Ts));
    N = samplesPerPeriod * numPeriods;   % total window length
    buffer = zeros(N, 1);
    sumBuf = 0;
    idx = 1;
    count = 0;          % number of samples received so far
end

% Update circular buffer: subtract oldest only if buffer is already full
if count >= N
    % Full window mode: subtract the sample that will be overwritten
    sumBuf = sumBuf - buffer(idx);
else
    % Startup mode: no subtraction, just accumulating
    % (buffer initially zeros, so subtracting would incorrectly remove zeros)
end

% Store new sample and update sum
buffer(idx) = u;
sumBuf = sumBuf + u;
idx = mod(idx, N) + 1;
count = count + 1;

% Output the average over the actual number of samples received so far
if count < N
    y = sumBuf / count;    % running average from first sample
else
    y = sumBuf / N;        % steady-state full‑window average
end
end

== matlab function ADC_SPWM_Openloop_2_Version_2/MATLAB Function5 ==
  data: u input; y output; f input; Ts input; numPeriods input
function y = dcOffset_EMA(u, f, Ts, numPeriods)
%#codegen
% Exponential moving average - C-friendly
% Time constant = numPeriods * (1/f)

persistent alpha y_prev

if isempty(alpha)
    samplesPerPeriod = round(1 / (f * Ts));
    N = samplesPerPeriod * numPeriods;
    alpha = 1 / N;
    y_prev = u;
end

% First-order low-pass filter
y = y_prev + alpha * (u - y_prev);
y_prev = y;
end

== matlab function ADC_SPWM_Openloop_2_Version_2/MATLAB Function6 ==
  data: u input; offset output; f input; Ts input; numPeriods input
function offset = dcOffset_Tracker(u, f, Ts, numPeriods)
%#codegen
% Speed-Adaptive DC Offset Tracker (Exponential Moving Average)
% Safely extracts DC offset from an AC signal using motor speed.

persistent y_prev

% --- Convert input to float to prevent ADC integer mismatch ---
% ADC blocks usually output uint16. We convert it to 'single' (float) 
% for safe math on DSPs without losing performance.
u_float = single(u);

% --- 1. Bumpless Initialization ---
% Start exactly at the first sampled value to prevent massive startup transients.
if isempty(y_prev)
    y_prev = u_float; 
end

% --- 2. Safe Frequency Handling ---
% Motor can spin backwards, so take the absolute value.
f_abs = abs(f);

% CRITICAL SAFETY: Prevent the "Zero-Speed Freeze".
% If the motor stops, we still want to track slow thermal drifts in the ADC.
% We enforce a minimum tracking frequency (e.g., 2.0 Hz).
f_min = 2.0; 
if f_abs < f_min
    f_effective = f_min;
else
    f_effective = f_abs;
end

% --- 3. Calculate Alpha (Safe Math) ---
% Original concept: time_constant = numPeriods * (1/f)
% By doing the algebra, Alpha = (f * Ts) / numPeriods
% This COMPLETELY ELIMINATES the division by frequency!
safe_numPeriods = max(numPeriods, 0.1); % Lowered to 0.1 to allow very fast tracking if desired
alpha = (f_effective * Ts) / safe_numPeriods;

% --- 4. Alpha Bounds (High-Speed Safety) ---
% At high frequencies (like 4000 Hz), alpha needs to be larger to track fast.
% We raise the clamp from 0.1 to 0.5. 
% (alpha = 0.5 means the new sample has 50% weight. Anything > 0.5 starts losing its filtering effect).
if alpha > .3
    alpha = .3;
end

% --- 5. Filter Update (Numerically Stable) ---
offset = y_prev + alpha * (u_float - y_prev);

% Store for the next cycle
y_prev = offset;

end

== matlab function ADC_SPWM_Openloop_2_Version_2/MATLAB Function7 ==
  data: u input; offset output; f input; Ts input; numPeriods input
function offset = dcOffset_Tracker(u, f, Ts, numPeriods)
%#codegen
% Speed-Adaptive DC Offset Tracker (Exponential Moving Average)
% OPTIMIZED FOR 4.5 kHz CONTROL LOOPS (Strict Single-Precision)

persistent y_prev

% --- 1. Strict Float Conversion ---
u_float = single(u);
f_float = single(f);
Ts_float = single(Ts);
numP_float = single(numPeriods);

% --- 2. Bumpless Initialization ---
if isempty(y_prev)
    y_prev = u_float; 
end

% --- 3. Safe Frequency Handling ---
f_abs = abs(f_float);

% Use single(2.0) to prevent double-precision math promotion!
f_min = single(2.0); 
if f_abs < f_min
    f_effective = f_min;
else
    f_effective = f_abs;
end

% --- 4. Calculate Alpha (Safe Math) ---
safe_numPeriods = max(numP_float, single(0.1)); 
alpha = (f_effective * Ts_float) / safe_numPeriods;

% --- 5. Alpha Bounds (High-Speed Safety) ---
if alpha > single(0.5)
    alpha = single(0.5);
end

% --- 6. Filter Update (Numerically Stable) ---
offset = y_prev + alpha * (u_float - y_prev);

% Store for the next cycle
y_prev = offset;

end

== matlab function ADC_SPWM_Openloop_2_Version_2/MATLAB Function9 ==
  data: u input; offset output; f input; Ts input; numPeriods input
function offset = dcOffset_Tracker(u, f, Ts, numPeriods)
%#codegen
% Speed-Adaptive DC Offset Tracker (Exponential Moving Average)
% OPTIMIZED FOR 4.5 kHz CONTROL LOOPS (Strict Single-Precision)

persistent y_prev

% --- 1. Strict Float Conversion ---
u_float = single(u);
f_float = single(f);
Ts_float = single(Ts);
numP_float = single(numPeriods);

% --- 2. Bumpless Initialization ---
if isempty(y_prev)
    y_prev = u_float; 
end

% --- 3. Safe Frequency Handling ---
f_abs = abs(f_float);

% Use single(2.0) to prevent double-precision math promotion!
f_min = single(2.0); 
if f_abs < f_min
    f_effective = f_min;
else
    f_effective = f_abs;
end

% --- 4. Calculate Alpha (Safe Math) ---
safe_numPeriods = max(numP_float, single(0.1)); 
alpha = (f_effective * Ts_float) / safe_numPeriods;

% --- 5. Alpha Bounds (High-Speed Safety) ---
if alpha > single(0.5)
    alpha = single(0.5);
end

% --- 6. Filter Update (Numerically Stable) ---
offset = y_prev + alpha * (u_float - y_prev);

% Store for the next cycle
y_prev = offset;

end
